simulink model "G_PF"  (R2018b)
settings: Solver=VariableStepAuto  StartTime=0.0  StopTime=10.0  RelTol=1e-3
undefined symbols (not defined in the file): T_gP, V_gPF
settings Model: Creator=rache  LastModifiedBy=rache

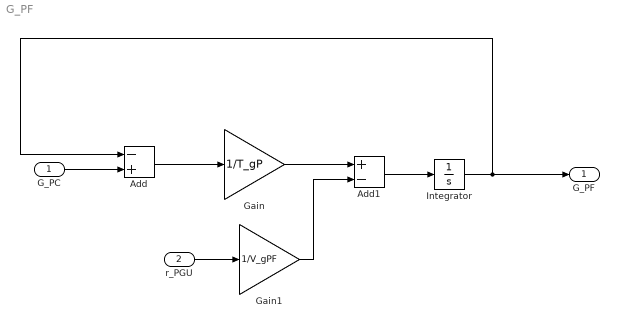
== system G_PF ==
  G_PC : Inport
  r_PGU : Inport  Port=2
  Add : Sum  Inputs=-+
  Add1 : Sum  Inputs=+-
  Gain : Gain  Gain=1/T_gP
  Gain1 : Gain  Gain=1/V_gPF
  Integrator : Integrator
  G_PF : Outport
  wires:
  Integrator/1 -> Add/1, G_PF/1
  G_PC/1 -> Add/2
  Add/1 -> Gain/1
  r_PGU/1 -> Gain1/1
  Gain1/1 -> Add1/2
  Gain/1 -> Add1/1
  Add1/1 -> Integrator/1
